simulink model "Simulink_pt1"  (R2020a)
settings: Solver=VariableStepAuto  StartTime=0.0  StopTime=10  RelTol=1e-3
libraries: simulink x2
settings Model: Creator=João Fernando Rangel  LastModifiedBy=João Fernando Rangel

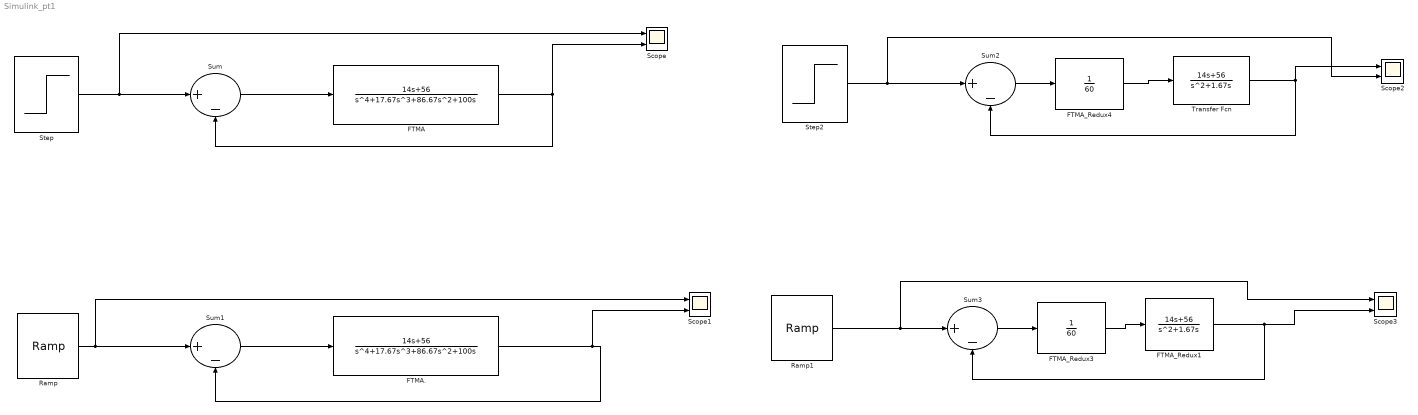
== system Simulink_pt1 ==
  FTMA : TransferFcn  Numerator=[0 0 0 0 14 56]  Denominator=[1 17.67 86.67 100 0]
  FTMA. : TransferFcn  Numerator=[0 0 0 0 14 56]  Denominator=[1 17.67 86.67 100 0]
  FTMA_Redux1 : TransferFcn  Tag=FTMA_Redux  Numerator=[14 56]  Denominator=[1 1.67 0]
  FTMA_Redux3 : TransferFcn  Tag=FTMA_Redux  Numerator=[0 1]  Denominator=[0 60]
  FTMA_Redux4 : TransferFcn  Tag=FTMA_Redux  Numerator=[0 1]  Denominator=[0 60]
  Ramp : simulink/Sources/Ramp  slope=1  start=0  InitialOutput=0
  Ramp1 : simulink/Sources/Ramp  slope=1  start=0  InitialOutput=0
  Scope{,1..3} (4 alike) : Scope  NumInputPorts=2
  Step : Step  Time=0  SampleTime=0
  Step2 : Step  Time=0  SampleTime=0
  Sum{,1..3} (4 alike) : Sum  Inputs=|+-
  Transfer Fcn : TransferFcn  Numerator=[0 14 56]  Denominator=[1 1.67 0]
  wires:
  Sum/1 -> FTMA/1
  FTMA/1 -> Scope/2, Sum/2
  Step/1 -> Scope/1, Sum/1
  FTMA./1 -> Scope1/2, Sum1/2
  Sum1/1 -> FTMA./1
  Ramp/1 -> Scope1/1, Sum1/1
  Ramp1/1 -> Scope3/1, Sum3/1
  Sum3/1 -> FTMA_Redux3/1
  FTMA_Redux3/1 -> FTMA_Redux1/1
  FTMA_Redux1/1 -> Scope3/2, Sum3/2
  Sum2/1 -> FTMA_Redux4/1
  FTMA_Redux4/1 -> Transfer Fcn/1
  Transfer Fcn/1 -> Scope2/1, Sum2/2
  Step2/1 -> Scope2/2, Sum2/1
